simulink model "DriveTrain_Modular"  (R2019a)
settings: Solver=VariableStepAuto  StartTime=0.0  StopTime=0.6  FixedStep=Ts  MinStep=Ts/5  RelTol=1e-3
InitFcn:
  | DriveTrainInitialise;
undefined symbols (not defined in the file or in its folder): J, ratio, RotorInertia, Ts, Vnom
libraries: fl_lib x3, nesl_utility x3, ee_lib x2, eeGeneralControl x2, dspfdesign x2, InverterLIB x1, MotorLIB x1
settings Model: OrderedModelArguments=off  Creator=plewi  LastModifiedBy=plewi
settings SolverCC: ZeroCrossAlgorithm=Adaptive
settings DataIOCC: SaveOutput=off  OutputTimes=SDO_OutputTimes  ReturnWorkspaceOutputsName=SDOSimTest_Log
settings DebuggingCC: IgnoredZcDiagnostic=none

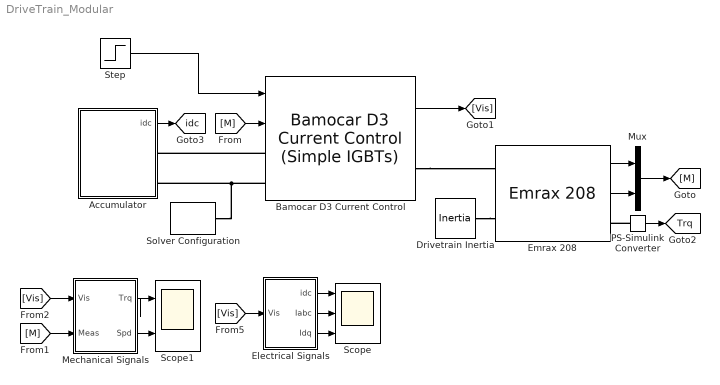
== system DriveTrain_Modular ==
  Accumulator : Subsystem  AncestorBlock=AccumulatorLIB/Accumulator (Simple)
  Bamocar D3 Current Control : InverterLIB/Bamocar D3 Current Control (Simple IGBTs)  Vnom=Vnom  Pmax=Pmax  Tmax=Tmax  Iq_max=80  p=PolePairs  Vdc_on=20  Ts=Ts  Tsc=Tsc  Ron=0.01  Goff=1e-8  Vf=0.5  diode_Vf=1.55  diode_Ron=0.01  diode_Goff=1e-8  RefType=Zero d-axis control  psim=PM  AxisAlignment=Q-axis  Kp_id=KdP  Ki_id=KdI  Kaw_id=KdAW  Kp_iq=KqP  Ki_iq=KqI  Kaw_iq=KqAW  AxisPrio=Q-axis  CPWMMode=SVM: space vector modulation  fsw=fsw
      settings: SamplingMode=Natural
  Drivetrain Inertia : fl_lib/Mechanical/Rotational Elements/Inertia  inertia=J*ratio kg*m^2  w_specify=off  w_priority=High  w=0 rad/s  w_nominal_specify=off  w_nominal_unit=rad/s  w_nominal_value=1  t_specify=off  t_priority=None  t=0 N*m  t_nominal_specify=off  t_nominal_unit=N*m  t_nominal_value=1
  Electrical Signals : Subsystem
  Emrax 208 : MotorLIB/Emrax 208  nPolePairs=PolePairs  pm_flux_linkage=PM  Ld=Ld  Lq=Lq  L0=2e-4  Rs=Rs  zero_sequence=ee.enum.park.zerosequence.exclude  J=RotorInertia  mask(Emrax 208){}
  Mechanical Signals : Subsystem
  Mux : Mux  Inputs=2
  PS-Simulink Converter : nesl_utility/PS-Simulink Converter  PhysicalDomain=network_engine_domain  SubClassName=ps_output  LeftPortType=input  RightPortType=output  PseudoPeriodic=off  Frequencies=[]  Unit=1  AffineConversion=off
  Scope : Scope  NumInputPorts=3
  Scope1 : Scope  NumInputPorts=2
  Solver Configuration : nesl_utility/Solver Configuration  PhysicalDomain=network_engine_domain  SubClassName=solver  LeftPortType=input  RightPortType=generic  Tones=[]  Harmonics=[]  SimulateNoise=off  Profile=off  UseLocalSampling=off  EnableSwitchedLinearOptims=on  FrequencyDomain=off  UseCCode=off  RelTol=0.001  AbsTol=1e-06  MinStep=1e-09  ToWorkspace=off  RevertToSquareIcSolve=off  NumHomotopyIterations=100  PhasorMode=off  PhasorModeNumHarmonics=1  DoDC=off  ResidualTolerance=1e-09  UseLocalSolver=off  LocalSolverChoice=NE_BACKWARD_EULER_ADVANCER  LocalSolverSampleTime=0.001  DoFixedCost=off  MaxNonlinIter=3  MaxModeIter=2  LinearAlgebra=auto  EquationFormulation=NE_TIME_EF  DelaysMemoryBudget=1024  AutomaticFiltering=on  FilteringTimeConstant=0.001  PartitionStorageMethod=AS_NEEDED  PartitionMemoryBudget=1024  PartitionMethod=ROBUST
  Step : Step  Time=0.1  After=20  SampleTime=0
      settings: AttributesFormatString=|
      | %<After> Nm at
      | %<Time>
  tag scope: Trq=global, idc=global
  wires:
  Mux/1 -> [M]
  [M] -> Bamocar D3 Current Control/2
  Emrax 208/1 -> Mux/1
  Emrax 208/2 -> Mux/2
  Bamocar D3 Current Control/1 -> [Vis]
  PS-Simulink Converter/1 -> [Trq]
  Accumulator/1(idc) -> [idc]
  Electrical Signals/1(idc) -> Scope/1
  Electrical Signals/3(Idq) -> Scope/3
  [M] -> Mechanical Signals/2("Meas ")
  [Vis] -> Mechanical Signals/1(Vis)
  Electrical Signals/2(Iabc) -> Scope/2
  Mechanical Signals/1(Trq) -> Scope1/1
  Mechanical Signals/2(Spd) -> Scope1/2
  [Vis] -> Electrical Signals/1(Vis)
  Step/1 -> Bamocar D3 Current Control/1
  connections:
  Bamocar D3 Current Control/LConn2 -- Solver Configuration/RConn1 -- Accumulator/RConn2
  PS-Simulink Converter/LConn1 -- Emrax 208/RConn1
  Bamocar D3 Current Control/LConn1 -- Accumulator/RConn1
  Bamocar D3 Current Control/RConn1 -- Emrax 208/LConn1
  Drivetrain Inertia/LConn1 -- Emrax 208/LConn2

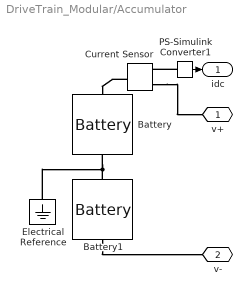
== system DriveTrain_Modular/Accumulator ==
  Battery : ee_lib/Sources/Battery  Vnom=Vnom/2 V  R1=0.001 Ohm  prm_AH=1  AH=14000 hr*A  V1=470 V  AH1=5000 hr*A  prm_R2=1  R2=inf Ohm  prm_dyn=1  Rp1=0.005 Ohm  tau1=30 s  Rp2=0.005 Ohm  tau2=30 s  Rp3=0.005 Ohm  tau3=30 s  Rp4=0.005 Ohm  tau4=30 s  Rp5=0.005 Ohm  tau5=30 s  prm_fade=1  N_fade=100  AH_fade=45 hr*A  R1_fade=2.02 Ohm  V1_fade=10.35 V  i_specify=off  i_priority=Low  i=0 A  i_nominal_specify=off  i_nominal_unit=A  i_nominal_value=1  v_specify=on  v_priority=High  v=Vnom/2 V  v_nominal_specify=off  v_nominal_unit=V  v_nominal_value=1  charge_specify=on  charge_priority=None  charge=7000 hr*A  charge_nominal_specify=off  charge_nominal_unit=hr*A  charge_nominal_value=1  num_cycles_specify=on  num_cycles_priority=None  num_cycles=0  num_cycles_nominal_specify=off  num_cycles_nominal_unit=1  num_cycles_nominal_value=1  thermal_mass=30000 J/K  Tmeas=298.15 K  Vnom_T2=12 V  R1_T2=2.2 Ohm  V1_T2=11.4 V  R2_T2=2200 Ohm  Rp1_T2=0.005 Ohm  tau1_T2=30 s  Rp2_T2=0.005 Ohm  tau2_T2=30 s  Rp3_T2=0.005 Ohm  tau3_T2=30 s  Rp4_T2=0.005 Ohm  tau4_T2=30 s  Rp5_T2=0.005 Ohm  tau5_T2=30 s  Tmeas2=273.15 K  temperature_specify=off  temperature_priority=High  temperature=298.15 K  temperature_nominal_specify=off  temperature_nominal_unit=K  temperature_nominal_value=1
      settings: SourceProductName=Simscape Electrical
  Battery1 : ee_lib/Sources/Battery  Vnom=Vnom/2 V  R1=0.001 Ohm  prm_AH=1  AH=14000 hr*A  V1=470 V  AH1=5000 hr*A  prm_R2=1  R2=inf Ohm  prm_dyn=1  Rp1=0.005 Ohm  tau1=30 s  Rp2=0.005 Ohm  tau2=30 s  Rp3=0.005 Ohm  tau3=30 s  Rp4=0.005 Ohm  tau4=30 s  Rp5=0.005 Ohm  tau5=30 s  prm_fade=1  N_fade=100  AH_fade=45 hr*A  R1_fade=2.02 Ohm  V1_fade=10.35 V  i_specify=off  i_priority=Low  i=0 A  i_nominal_specify=off  i_nominal_unit=A  i_nominal_value=1  v_specify=on  v_priority=High  v=Vnom/2 V  v_nominal_specify=off  v_nominal_unit=V  v_nominal_value=1  charge_specify=on  charge_priority=None  charge=7000 hr*A  charge_nominal_specify=off  charge_nominal_unit=hr*A  charge_nominal_value=1  num_cycles_specify=on  num_cycles_priority=None  num_cycles=0  num_cycles_nominal_specify=off  num_cycles_nominal_unit=1  num_cycles_nominal_value=1  thermal_mass=30000 J/K  Tmeas=298.15 K  Vnom_T2=12 V  R1_T2=2.2 Ohm  V1_T2=11.4 V  R2_T2=2200 Ohm  Rp1_T2=0.005 Ohm  tau1_T2=30 s  Rp2_T2=0.005 Ohm  tau2_T2=30 s  Rp3_T2=0.005 Ohm  tau3_T2=30 s  Rp4_T2=0.005 Ohm  tau4_T2=30 s  Rp5_T2=0.005 Ohm  tau5_T2=30 s  Tmeas2=273.15 K  temperature_specify=off  temperature_priority=High  temperature=298.15 K  temperature_nominal_specify=off  temperature_nominal_unit=K  temperature_nominal_value=1
      settings: SourceProductName=Simscape Electrical
  Current Sensor : fl_lib/Electrical/Electrical Sensors/Current Sensor
  Electrical Reference : fl_lib/Electrical/Electrical Elements/Electrical Reference
      settings: SourceProductName=Foundation Library
  PS-Simulink Converter1 : nesl_utility/PS-Simulink Converter  PhysicalDomain=network_engine_domain  SubClassName=ps_output  LeftPortType=input  RightPortType=output  PseudoPeriodic=off  Frequencies=[]  Unit=1  AffineConversion=off
  v+ : PMIOPort  Side=Right
  v- : PMIOPort  Port=2  Side=Right
  idc : Outport
  wires:
  PS-Simulink Converter1/1 -> idc/1
  connections:
  Battery1/RConn1 -- v-/RConn1
  PS-Simulink Converter1/LConn1 -- Current Sensor/RConn1
  Current Sensor/RConn2 -- v+/RConn1
  Current Sensor/LConn1 -- Battery/LConn1
  Battery1/LConn1 -- Electrical Reference/LConn1 -- Battery/RConn1

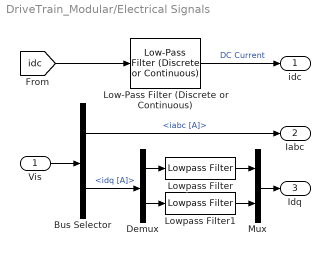
== system DriveTrain_Modular/Electrical Signals ==
  Vis : Inport
  Bus Selector : BusSelector  OutputSignals=signal2.iabc [A],signal2.idq [A]
  Demux : Demux  Outputs=2
  Low-Pass Filter (Discrete or Continuous) : eeGeneralControl/Low-Pass Filter (Discrete or Continuous)  K=1  T=0.04  B=inf  A=-inf  Ts=-1
      settings: SourceProductName=Simscape Electrical
  Lowpass Filter : dspfdesign/Lowpass Filter  FilterType=IIR  DesignForMinimumOrder=on  FilterOrder=50  PassbandFrequency=8e2  StopbandFrequency=12e3  PassbandRipple=0.1  StopbandAttenuation=80  InheritSampleRate=off  SampleRate=44100  SimulateUsing=Interpreted execution  roundingMode=Floor  coeffsDataTypeStr=fixdt(1,16)
  Lowpass Filter1 : dspfdesign/Lowpass Filter  FilterType=IIR  DesignForMinimumOrder=on  FilterOrder=50  PassbandFrequency=8e2  StopbandFrequency=12e3  PassbandRipple=0.1  StopbandAttenuation=80  InheritSampleRate=off  SampleRate=44100  SimulateUsing=Interpreted execution  roundingMode=Floor  coeffsDataTypeStr=fixdt(1,16)
  Mux : Mux  Inputs=2
  idc : Outport
  Iabc : Outport  Port=2
  Idq : Outport  Port=3
  wires:
  Low-Pass Filter (Discrete or Continuous)/1 -> idc/1  "DC Current"
  [idc] -> Low-Pass Filter (Discrete or Continuous)/1
  Vis/1 -> Bus Selector/1
  Bus Selector/1 -> Iabc/1  "<iabc [A]>"
  Bus Selector/2 -> Demux/1  "<idq [A]>"
  Demux/1 -> Lowpass Filter/1
  Lowpass Filter/1 -> Mux/1
  Mux/1 -> Idq/1
  Demux/2 -> Lowpass Filter1/1
  Lowpass Filter1/1 -> Mux/2

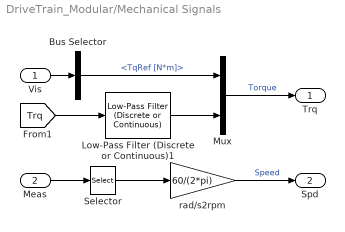
== system DriveTrain_Modular/Mechanical Signals ==
  Vis : Inport
  "Meas " : Inport  Port=2
  Bus Selector : BusSelector  OutputSignals=signal2.TqRef [N*m]
  Low-Pass Filter (Discrete or Continuous)1 : eeGeneralControl/Low-Pass Filter (Discrete or Continuous)  K=1  T=4e-2  B=inf  A=-inf  Ts=-1
      settings: SourceProductName=Simscape Electrical
  Mux : Mux  Inputs=2
  Selector : Selector  InputPortWidth=2  IndexOptions=Index vector (dialog)  Indices=[1]  OutputSizes=1
  rad/s2rpm : Gain  Gain=60/(2*pi)
  Trq : Outport
  Spd : Outport  Port=2
  wires:
  Vis/1 -> Bus Selector/1
  rad/s2rpm/1 -> Spd/1  "Speed"
  Selector/1 -> rad/s2rpm/1
  Mux/1 -> Trq/1  "Torque"
  Bus Selector/1 -> Mux/1  "<TqRef [N*m]>"
  "Meas "/1 -> Selector/1
  [Trq] -> Low-Pass Filter (Discrete or Continuous)1/1
  Low-Pass Filter (Discrete or Continuous)1/1 -> Mux/2
